simulink model "QuadcopterLinearZero"  (R2020a)
settings: Solver=VariableStepAuto  StartTime=0.0  StopTime=10.0  RelTol=1e-3
undefined symbols (not defined in the file or in its folder): A1, A3, B1, B3, C2
settings Model: Creator=Ali  LastModifiedBy=Ali

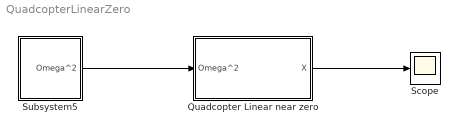
== system QuadcopterLinearZero ==
  Quadcopter Linear near zero : Subsystem
      mask Display: image('E:\Control\Quadcopter\drone_PNG203.png'); % Use "Edit Image" on toolstrip to change.
  Scope : Scope
  Subsystem5 : Subsystem
  wires:
  Subsystem5/1(Omega^2) -> Quadcopter Linear near zero/1(Omega^2)
  Quadcopter Linear near zero/1(X) -> Scope/1

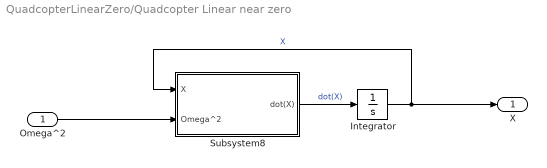
== system QuadcopterLinearZero/Quadcopter Linear near zero ==
  Omega^2 : Inport
  Integrator : Integrator
  Subsystem8 : Subsystem
  X : Outport
  wires:
  Integrator/1 -> X/1, Subsystem8/1(X)  "X"
  Subsystem8/1(dot(X)) -> Integrator/1  "dot(X)"
  Omega^2/1 -> Subsystem8/2(Omega^2)

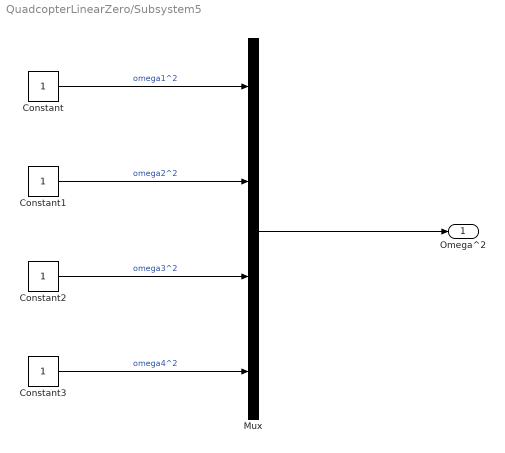
== system QuadcopterLinearZero/Subsystem5 ==
  Constant{,1..3} (4 alike) : Constant
  Mux : Mux
  Omega^2 : Outport
  wires:
  Constant1/1 -> Mux/2  "omega2^2"
  Constant2/1 -> Mux/3  "omega3^2"
  Constant3/1 -> Mux/4  "omega4^2"
  Constant/1 -> Mux/1  "omega1^2"
  Mux/1 -> Omega^2/1

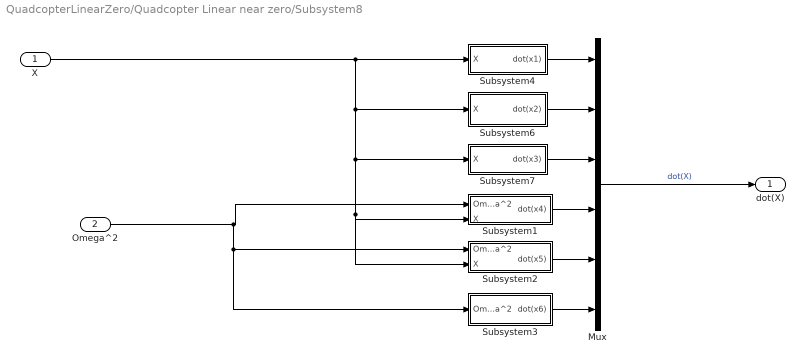
== system QuadcopterLinearZero/Quadcopter Linear near zero/Subsystem8 ==
  X : Inport
  Omega^2 : Inport  Port=2
  Mux : Mux  Inputs=6
  Subsystem1 : Subsystem
  Subsystem2 : Subsystem
  Subsystem3 : Subsystem
  Subsystem4 : Subsystem
  Subsystem6 : Subsystem
  Subsystem7 : Subsystem
  dot(X) : Outport
  wires:
  Omega^2/1 -> Subsystem2/1(Omega^2), Subsystem3/1(Omega^2), Subsystem1/1(Omega^2)
  Subsystem3/1(dot(x6)) -> Mux/6
  Subsystem7/1(dot(x3)) -> Mux/3
  Subsystem1/1(dot(x4)) -> Mux/4
  Subsystem6/1(dot(x2)) -> Mux/2
  X/1 -> Subsystem2/2(X), Subsystem1/2(X), Subsystem7/1(X), Subsystem6/1(X), Subsystem4/1(X)
  Subsystem2/1(dot(x5)) -> Mux/5
  Subsystem4/1(dot(x1)) -> Mux/1
  Mux/1 -> dot(X)/1  "dot(X)"

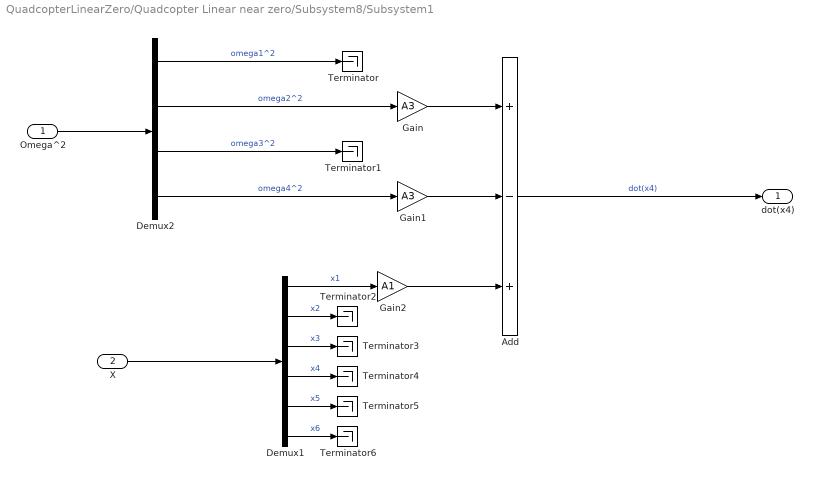
== system QuadcopterLinearZero/Quadcopter Linear near zero/Subsystem8/Subsystem1 ==
  Omega^2 : Inport
  X : Inport  Port=2
  Add : Sum  Inputs=+-+
  Demux1 : Demux  Outputs=6
  Demux2 : Demux
  Gain : Gain  Gain=A3
  Gain1 : Gain  Gain=A3
  Gain2 : Gain  Gain=A1
  Terminator{,1..6} (7 alike) : Terminator
  dot(x4) : Outport
  wires:
  Gain2/1 -> Add/3
  Gain1/1 -> Add/2
  Add/1 -> dot(x4)/1  "dot(x4)"
  Gain/1 -> Add/1
  Demux2/4 -> Gain1/1  "omega4^2"
  Demux2/2 -> Gain/1  "omega2^2"
  Demux2/3 -> Terminator1/1  "omega3^2"
  Demux2/1 -> Terminator/1  "omega1^2"
  Omega^2/1 -> Demux2/1
  Demux1/5 -> Terminator5/1  "x5"
  Demux1/2 -> Terminator2/1  "x2"
  Demux1/3 -> Terminator3/1  "x3"
  Demux1/1 -> Gain2/1  "x1"
  Demux1/4 -> Terminator4/1  "x4"
  X/1 -> Demux1/1
  Demux1/6 -> Terminator6/1  "x6"

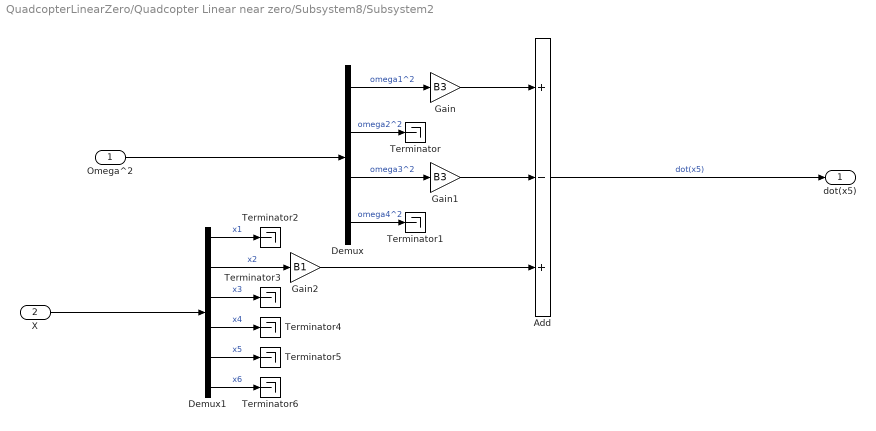
== system QuadcopterLinearZero/Quadcopter Linear near zero/Subsystem8/Subsystem2 ==
  Omega^2 : Inport
  X : Inport  Port=2
  Add : Sum  Inputs=+-+
  Demux : Demux
  Demux1 : Demux  Outputs=6
  Gain : Gain  Gain=B3
  Gain1 : Gain  Gain=B3
  Gain2 : Gain  Gain=B1
  Terminator{,1..6} (7 alike) : Terminator
  dot(x5) : Outport
  wires:
  Gain2/1 -> Add/3
  Gain1/1 -> Add/2
  Add/1 -> dot(x5)/1  "dot(x5)"
  Gain/1 -> Add/1
  Omega^2/1 -> Demux/1
  Demux/2 -> Terminator/1  "omega2^2"
  Demux/4 -> Terminator1/1  "omega4^2"
  Demux/1 -> Gain/1  "omega1^2"
  Demux/3 -> Gain1/1  "omega3^2"
  Demux1/5 -> Terminator5/1  "x5"
  Demux1/2 -> Gain2/1  "x2"
  Demux1/3 -> Terminator3/1  "x3"
  Demux1/1 -> Terminator2/1  "x1"
  Demux1/4 -> Terminator4/1  "x4"
  X/1 -> Demux1/1
  Demux1/6 -> Terminator6/1  "x6"

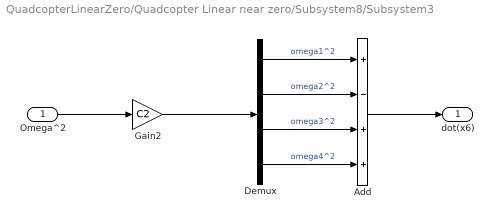
== system QuadcopterLinearZero/Quadcopter Linear near zero/Subsystem8/Subsystem3 ==
  Omega^2 : Inport
  Add : Sum  Inputs=+-++
  Demux : Demux
  Gain2 : Gain  Gain=C2
  dot(x6) : Outport
  wires:
  Omega^2/1 -> Gain2/1
  Gain2/1 -> Demux/1
  Demux/1 -> Add/1  "omega1^2"
  Demux/2 -> Add/2  "omega2^2"
  Demux/3 -> Add/3  "omega3^2"
  Demux/4 -> Add/4  "omega4^2"
  Add/1 -> dot(x6)/1

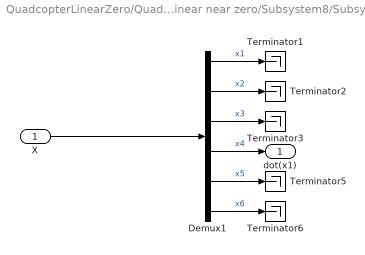
== system QuadcopterLinearZero/Quadcopter Linear near zero/Subsystem8/Subsystem4 ==
  X : Inport
  Demux1 : Demux  Outputs=6
  Terminator{1..3,5..6} (5 alike) : Terminator
  dot(x1) : Outport
  wires:
  Demux1/4 -> dot(x1)/1  "x4"
  X/1 -> Demux1/1
  Demux1/6 -> Terminator6/1  "x6"
  Demux1/5 -> Terminator5/1  "x5"
  Demux1/3 -> Terminator3/1  "x3"
  Demux1/2 -> Terminator2/1  "x2"
  Demux1/1 -> Terminator1/1  "x1"

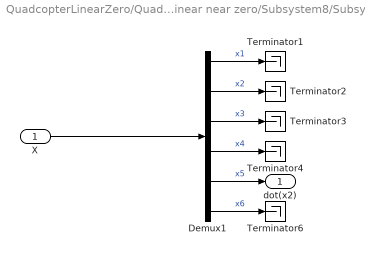
== system QuadcopterLinearZero/Quadcopter Linear near zero/Subsystem8/Subsystem6 ==
  X : Inport
  Demux1 : Demux  Outputs=6
  Terminator{1..4,6} (5 alike) : Terminator
  dot(x2) : Outport
  wires:
  Demux1/4 -> Terminator4/1  "x4"
  X/1 -> Demux1/1
  Demux1/6 -> Terminator6/1  "x6"
  Demux1/5 -> dot(x2)/1  "x5"
  Demux1/3 -> Terminator3/1  "x3"
  Demux1/2 -> Terminator2/1  "x2"
  Demux1/1 -> Terminator1/1  "x1"

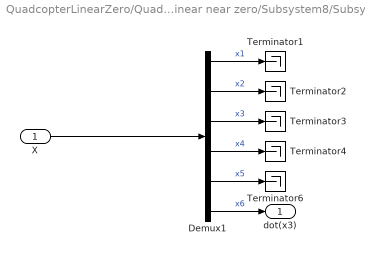
== system QuadcopterLinearZero/Quadcopter Linear near zero/Subsystem8/Subsystem7 ==
  X : Inport
  Demux1 : Demux  Outputs=6
  Terminator{1..4,6} (5 alike) : Terminator
  dot(x3) : Outport
  wires:
  Demux1/4 -> Terminator4/1  "x4"
  X/1 -> Demux1/1
  Demux1/6 -> dot(x3)/1  "x6"
  Demux1/5 -> Terminator6/1  "x5"
  Demux1/3 -> Terminator3/1  "x3"
  Demux1/2 -> Terminator2/1  "x2"
  Demux1/1 -> Terminator1/1  "x1"
